simulink model "Simulink_1"  (R2024b)
settings: Solver=ode4  StartTime=0.0  StopTime=130  FixedStep=0.01  RelTol=1e-3
values from neighbouring files (symbols this model uses):
  g = 9.81    [longMov.m]    (also in resistencias.m)
  M = 1020    [longMov.m]    (also in resistencias.m)
libraries: autolibshared x1
settings Model: Creator=caugu  LastModifiedBy=caugu

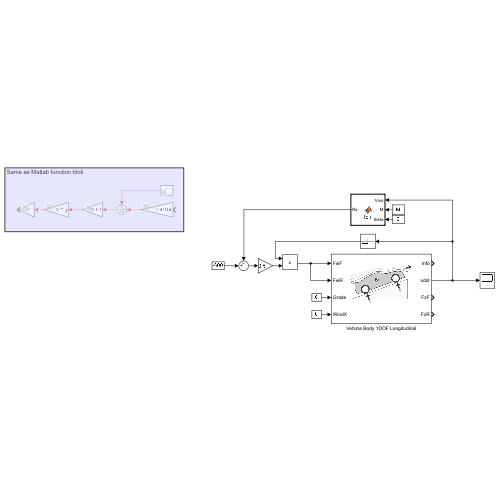
[thumbnail: Simulink's stored preview of the top-level diagram]
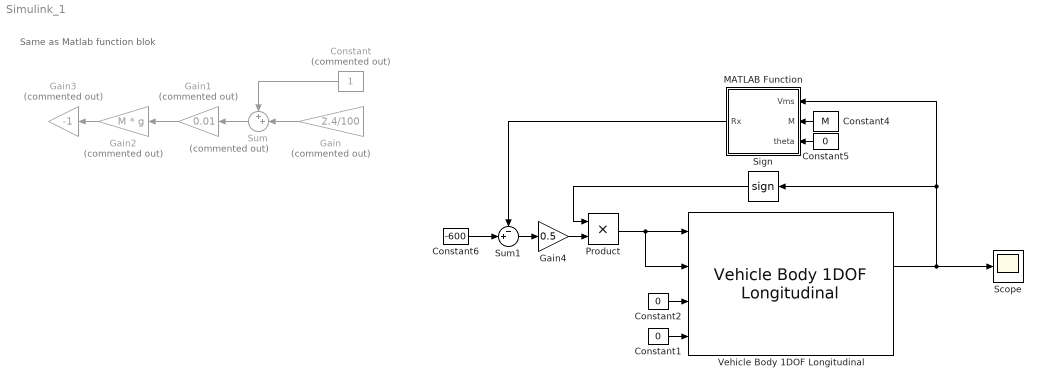
== system Simulink_1 ==
  note: Same as Matlab function blok
  Constant : Constant  Commented=on
  Constant1 : Constant  Value=0
  Constant2 : Constant  Value=0
  Constant4 : Constant  Value=M
  Constant5 : Constant  Value=0
  Constant6 : Constant  Value=-600
  Gain : Gain  Commented=on  Gain=2.4/100
  Gain1 : Gain  Commented=on  Gain=0.01
  Gain2 : Gain  Commented=on  Gain=M * g
  Gain3 : Gain  Commented=on  Gain=-1
  Gain4 : Gain  Gain=0.5
  MATLAB Function : MATLAB Function  TreatAsAtomicUnit=on
  Product : Product
  Scope : Scope
  Sign : Signum
  Sum : Sum  Commented=on  Inputs=++|
  Sum1 : Sum  Inputs=-+|
  Vehicle Body 1DOF Longitudinal : autolibshared/Vehicle Body 1DOF Longitudinal  VariantControl=SL  extFMode=off  extMMode=off  extTamb=off  wind3D=off  aMode=1  NF=2  NR=2  m=M  a=1.4  b=1.8  h=.35  Cd=.3  Cl=0  Cpm=0  Af=Af  x_o=0  xdot_o=80 / 3.6  Pabs=101325  T=273  g=9.81
      settings: LibrarySourceBlock=autolibvehdynlong/Vehicle Body 1DOF Longitudinal
  wires:
  Constant1/1 -> Vehicle Body 1DOF Longitudinal/4
  Vehicle Body 1DOF Longitudinal/2 -> Sign/1, MATLAB Function/1(Vms), Scope/1
  Constant2/1 -> Vehicle Body 1DOF Longitudinal/3
  Gain/1 -> Sum/2
  Constant/1 -> Sum/1
  Sum/1 -> Gain1/1
  Gain1/1 -> Gain2/1
  Gain2/1 -> Gain3/1
  Constant4/1 -> MATLAB Function/2(M)
  Constant5/1 -> MATLAB Function/3(theta)
  MATLAB Function/1(Rx) -> Sum1/1
  Constant6/1 -> Sum1/2
  Sum1/1 -> Gain4/1
  Gain4/1 -> Product/2
  Product/1 -> Vehicle Body 1DOF Longitudinal/2, Vehicle Body 1DOF Longitudinal/1
  Sign/1 -> Product/1

== matlab function Simulink_1/MATLAB Function ==
  data: Vms input; Rx output; M input; theta input
function Rx = fcn(Vms, M, theta)
g = 9.81;

% Coef. de Resistencia ao Rolamento:
W = M * g;

fr = 0.01 * (1 + (2.24 / 100) * Vms);
% Resistencia ao rolamento:
Rx = fr * W * cos(theta) * sign(Vms);       % [N]
